simulink model "Hunter_gazebo_call"  (R2023a)
settings: Solver=ode3  StartTime=0.0  StopTime=inf  FixedStep=0.05  RelTol=1e-3  EnableMultiTasking=on
InitFcn:
  | rosshutdown
  | rosinit("http://localhost:11311")
model workspace (MAT data in the model file):
  SL_ROS_VariableLengthArrays_MaxSizes.CommonInfo.ArrayTruncateAction = 'EmitWarning'
  SL_ROS_VariableLengthArrays_MaxSizes.MsgTypeMap = containers.Map
  SL_ROS_VariableLengthArrays_MaxSizes.MsgTypeMap.serialization.keys = {'cob_object_detection_msgs/Detection', 'cob_object_detection_msgs/DetectionArray', 'gazebo_msgs/ModelStates', 'sensor_msgs/PointCloud2'}
  SL_ROS_VariableLengthArrays_MaxSizes.MsgTypeMap.serialization.values{1}(1).PropertyName = 'Detector'
  SL_ROS_VariableLengthArrays_MaxSizes.MsgTypeMap.serialization.values{1}(1).DataType = 'uint8'
  SL_ROS_VariableLengthArrays_MaxSizes.MsgTypeMap.serialization.values{1}(1).MaxLength = 128
  SL_ROS_VariableLengthArrays_MaxSizes.MsgTypeMap.serialization.values{1}(2).PropertyName = 'Label'
  SL_ROS_VariableLengthArrays_MaxSizes.MsgTypeMap.serialization.values{1}(2).DataType = 'uint8'
  SL_ROS_VariableLengthArrays_MaxSizes.MsgTypeMap.serialization.values{1}(2).MaxLength = 128
  SL_ROS_VariableLengthArrays_MaxSizes.MsgTypeMap.serialization.values{2}.PropertyName = 'Detections'
  SL_ROS_VariableLengthArrays_MaxSizes.MsgTypeMap.serialization.values{2}.DataType = 'cob_object_detection_msgs/Detection'
  SL_ROS_VariableLengthArrays_MaxSizes.MsgTypeMap.serialization.values{2}.MaxLength = 100
  SL_ROS_VariableLengthArrays_MaxSizes.MsgTypeMap.serialization.values{3}(1).PropertyName = 'Name'
  SL_ROS_VariableLengthArrays_MaxSizes.MsgTypeMap.serialization.values{3}(1).DataType = 'std_msgs/String'
  SL_ROS_VariableLengthArrays_MaxSizes.MsgTypeMap.serialization.values{3}(1).MaxLength = 266
  SL_ROS_VariableLengthArrays_MaxSizes.MsgTypeMap.serialization.values{3}(2).PropertyName = 'Pose'
  SL_ROS_VariableLengthArrays_MaxSizes.MsgTypeMap.serialization.values{3}(2).DataType = 'geometry_msgs/Pose'
  SL_ROS_VariableLengthArrays_MaxSizes.MsgTypeMap.serialization.values{3}(2).MaxLength = 350
  SL_ROS_VariableLengthArrays_MaxSizes.MsgTypeMap.serialization.values{3}(3).PropertyName = 'Twist'
  SL_ROS_VariableLengthArrays_MaxSizes.MsgTypeMap.serialization.values{3}(3).DataType = 'geometry_msgs/Twist'
  SL_ROS_VariableLengthArrays_MaxSizes.MsgTypeMap.serialization.values{3}(3).MaxLength = 350
  SL_ROS_VariableLengthArrays_MaxSizes.MsgTypeMap.serialization.values{4}(1).PropertyName = 'Data'
  SL_ROS_VariableLengthArrays_MaxSizes.MsgTypeMap.serialization.values{4}(1).DataType = 'uint8'
  SL_ROS_VariableLengthArrays_MaxSizes.MsgTypeMap.serialization.values{4}(1).MaxLength = 1050000
  SL_ROS_VariableLengthArrays_MaxSizes.MsgTypeMap.serialization.values{4}(2).PropertyName = 'Fields'
  SL_ROS_VariableLengthArrays_MaxSizes.MsgTypeMap.serialization.values{4}(2).DataType = 'sensor_msgs/PointField'
  SL_ROS_VariableLengthArrays_MaxSizes.MsgTypeMap.serialization.values{4}(2).MaxLength = 1000
  SL_ROS_VariableLengthArrays_MaxSizes.MsgTypeMap.serialization.uniformity = 0
  SL_ROS_VariableLengthArrays_MaxSizes.MsgTypeMap.serialization.keyType = 'char'
  SL_ROS_VariableLengthArrays_MaxSizes.MsgTypeMap.serialization.valueType = 'any'
values from neighbouring files (symbols this model uses):
  roi = [0, 7, -7, 7, -1, 2]    [TrackExample_sim.m]
undefined symbols (not defined in the file or in its folder): Angular, L, Ld, Linear
libraries: robotlib x20, slpidlib x4, robotalgslib x3, slctrlblks x2, mobileRoboticsLib x2, robotcorelib x2, simulink_extras x2
(part 1 of 2)
settings Model: Creator=aiv_  LastModifiedBy=aiv
settings SolverCC: AutoInsertRateTranBlk=on
settings DataIOCC: SaveFormat=Array  ReturnWorkspaceOutputs=off
settings OptimizationCC: EnhancedBackFolding=on  PassReuseOutputArgsAs=Individual arguments  StateBitsets=on  DataBitsets=on  ZeroExternalMemoryAtStartup=off  ZeroInternalMemoryAtStartup=off  NoFixptDivByZeroProtection=on  LifeSpan=1  MaxStackSize=64  OptimizeBlockOrder=speed  DifferentSizesBufferReuse=on  EfficientTunableParamExpr=on
settings DebuggingCC: ParameterTunabilityLossMsg=error
settings HardwareCC: ProdBitPerPointer=32  ProdBitPerSizeT=32  ProdBitPerPtrDiffT=32  ProdLargestAtomicFloat=None  ProdWordSize=32  ProdHWDeviceType=Custom Processor->Custom Processor
settings ModelReferenceCC: PropagateSignalLabelsOutOfModel=off
settings SFSimCC: SimTargetLang=C++
settings RTWCC: Description=Embedded Coder  SystemTargetFile=ert.tlc  HardwareBoard=Robot Operating System (ROS)  TLCOptions=-p0 -aRateBasedStepFcn=0  TemplateMakefile=ert_default_tmf  GenerateReport=on  RTWVerbose=off  Toolchain=Catkin  IncludeHyperlinkInReport=on  LaunchReport=on  TargetLang=C++
settings CodeAppCC: ForceParamTrailComments=on  IgnoreCustomStorageClasses=off  OperatorAnnotations=on  SimulinkDataObjDesc=on  SFDataObjDesc=on  CustomSymbolStrGlobalVar=rt$N$M  CustomSymbolStrType=$N$M  CustomSymbolStrFcn=$N$M$F  CustomSymbolStrMacro=$N$M  InsertBlockDesc=on
settings ERTTargetCC: CodeReplacementLibrary=GNU C99 extensions  SuppressErrorStatus=on  CodeInterfacePackaging=C++ class  SupportVariableSizeSignals=on  RootIOFormat=Structure reference  ERTCustomFileTemplate=example_file_process.tlc

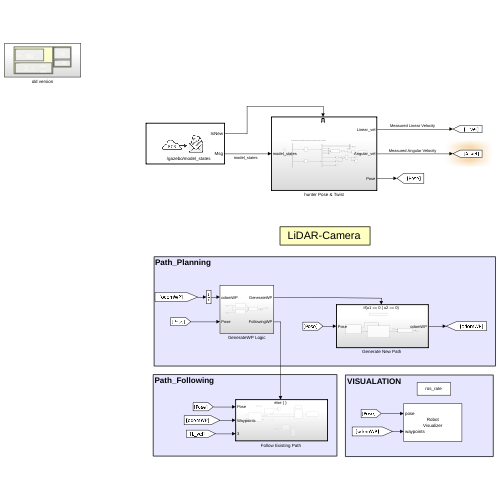
[thumbnail: Simulink's stored preview of the top-level diagram]
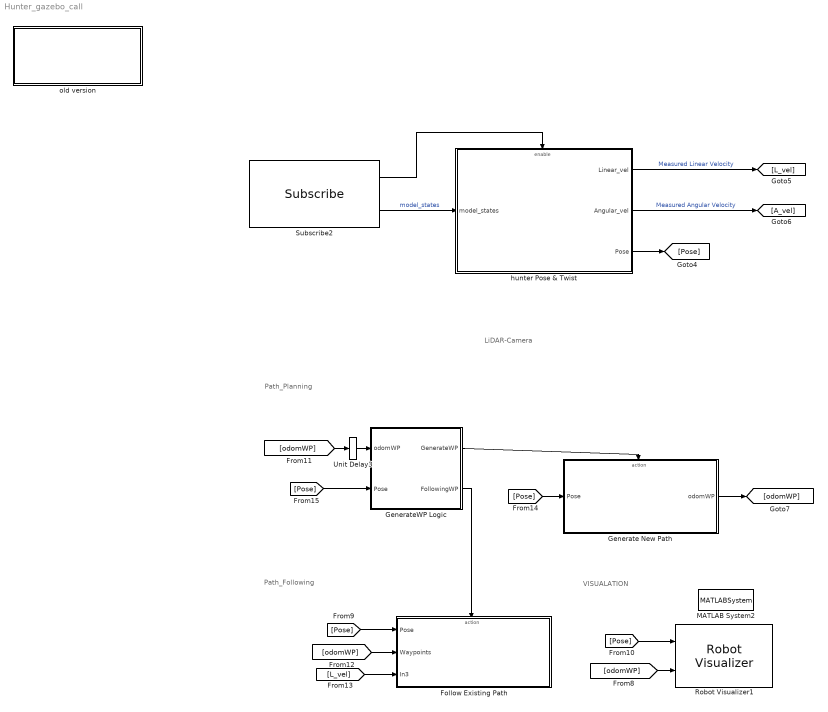
== system Hunter_gazebo_call ==
  note: LiDAR-Camera
  note: VISUALATION
  note: Path_Planning
  note: Path_Following
  "Follow Existing Path " : Subsystem  TreatAsAtomicUnit=on
  "Generate New Path " : Subsystem  TreatAsAtomicUnit=on
  GenerateWP Logic : Subsystem
  MATLAB System2 : MATLABSystem  System=ros_rate  RATE=[20]  SimulateUsing=Code generation
      mask Type: ros_rate
      mask Display: disp('ros_rate');
  Robot Visualizer1 : mobileRoboticsLib/Environments/Robot Visualizer  robotRadius=0  showTrajectory=on  hasWaypoints=on  hasLidar=off  sensorOffset=[ 0, 0 ]  scanAngles=[ -pi/4, 0, pi/4 ]  hasObjDetector=off  objDetectorOffset=[ 0, 0 ]  objDetectorAngle=0  objDetectorFOV=pi/4  objDetectorMaxRange=5  objectColors=[ 1, 0, 0; 0, 1, 0; 0, 0, 1 ]  objectMarkers=s
  Subscribe2 : robotlib/Subscribe  topicSource=Select from ROS network  topic=/gazebo/model_states  messageType=gazebo_msgs/ModelStates  SampleTime=-1  legacyBusStruct=off  messageQueueLength=1
  Unit Delay3 : UnitDelay  SampleTime=-1  HasFrameUpgradeWarning=on
  hunter Pose & Twist : Subsystem
  old version : Subsystem
  wires:
  hunter Pose & Twist/3(Pose) -> [Pose]
  Subscribe2/1 -> hunter Pose & Twist/Enable
  hunter Pose & Twist/2(Angular_vel) -> [A_vel]  "Measured Angular Velocity"
  Subscribe2/2 -> hunter Pose & Twist/1(model_states)  "model_states"
  hunter Pose & Twist/1(Linear_vel) -> [L_vel]  "Measured Linear Velocity"
  [odomWP] -> Robot Visualizer1/2
  [Pose] -> "Follow Existing Path "/1(Pose)
  "Generate New Path "/1(odomWP) -> [odomWP]
  [odomWP] -> "Follow Existing Path "/2(Waypoints)
  [Pose] -> GenerateWP Logic/2(Pose)
  [odomWP] -> Unit Delay3/1
  [Pose] -> "Generate New Path "/1(Pose)
  GenerateWP Logic/2(FollowingWP) -> "Follow Existing Path "/Action
  [Pose] -> Robot Visualizer1/1
  GenerateWP Logic/1(GenerateWP) -> "Generate New Path "/Action
  Unit Delay3/1 -> GenerateWP Logic/1(odomWP)
  [L_vel] -> "Follow Existing Path "/3(In3)

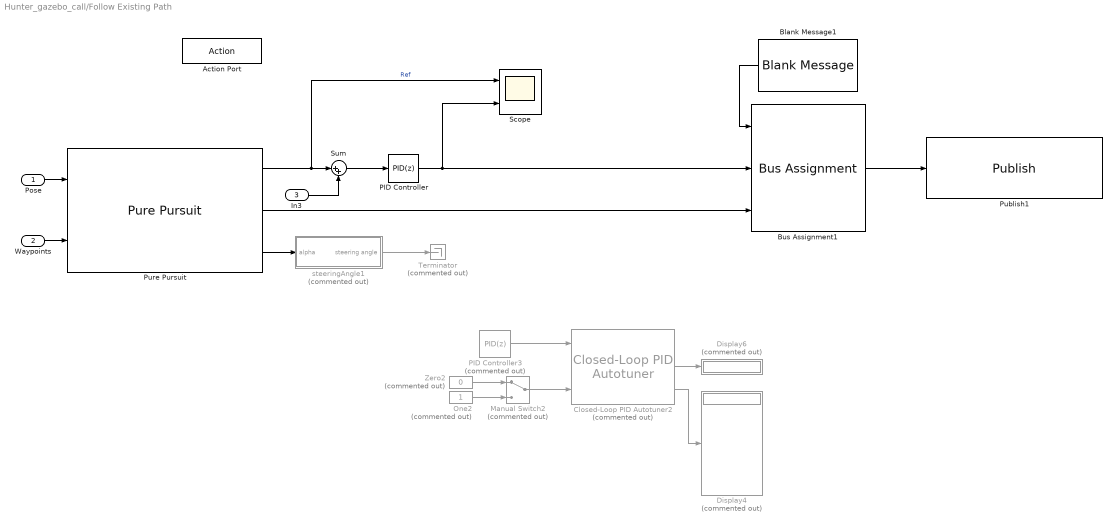
== system Hunter_gazebo_call/Follow Existing Path  ==
  Pose : Inport
  Waypoints : Inport  Port=2
  In3 : Inport  Port=3
  Action Port : ActionPort  ActionPortLabel=else
  Blank Message1 : robotlib/Blank Message  messageClass=Message  entityType=geometry_msgs/Twist  messageType=geometry_msgs/Twist  SampleTime=inf  legacyBusStruct=off
  Bus Assignment1 : BusAssignment  AssignedSignals=Linear.X,Angular.Z
  Closed-Loop PID Autotuner2 : slctrlblks/Closed-Loop PID Autotuner  Commented=on  PIDType=PID  PIDForm=Parallel  TimeDomain=discrete-time  DiscreteTs=0.05  TuningTs=0.2  UseTuningTs=off  IntegratorFormula=Forward Euler  FilterFormula=Forward Euler  ContinuousTs=0.02  Bandwidth=1  UseExternalWC=off  TargetPM=60  UseExternalPM=off  UseExternalAchievedPM=off  ExperimentMode=Superposition  PlantType=Stable  PlantSign=Positive  AmpSine=0.01  UseExternalAmpSine=off  UseExternalFRD=off  UseExternalU0=off  UseCompanion=off  NotDeployTuningModule=off  UsePLCCoder=off  OutputMode=control action + perturbation  BlockDataType=double  UseConnectedPID=on  blockpath=[]  tunedP=0  tunedI=0  tunedD=0  tunedN=100  tunedPM=0  EstimationWindowSize=3  UseExternalTuningParams=off  SingleMultiRateVariant=SingleSamplingRate  NumEstimationPeriods=4  NumSettlingPeriods=2  ExperimentModeVariant=VariantSuperimposed  OutputChoice=VariantCandD
  Display4 : Display  Commented=on
  Display6 : Display  Commented=on
  Manual Switch2 : ManualSwitch  Commented=on
  One2 : Constant  Commented=on  OutDataTypeStr=Inherit: Inherit via back propagation
  PID Controller : slpidlib/PID Controller  Controller=PID  Form=Parallel  TimeDomain=Discrete-time  UseExternalTs=off  SampleTime=-1  IntegratorMethod=Forward Euler  FilterMethod=Forward Euler  ControllerParametersSource=internal  P=0.3475  I=0.1757  UseKiTs=off  D=0  N=100  UseFilter=on  TunerSelectOption=Transfer Function Based (PID Tuner App)  InitialConditionSource=internal  InitialConditionForIntegrator=0  InitialConditionForFilter=0  DifferentiatorICPrevScaledInput=0  ExternalReset=none  TrackingMode=off  Kt=1  LimitOutput=off  SatLimitsSource=internal  UpperSaturationLimit=inf  LowerSaturationLimit=-inf  LinearizeAsGain=on  AntiWindupMode=none  Kb=1  LimitIntegrator=off  UpperIntegratorSaturationLimit=inf  LowerIntegratorSaturationLimit=-inf  POutMin=[]  POutMax=[]  IOutMin=[]  IOutMax=[]  DOutMin=[]  DOutMax=[]  NOutMin=[]  NOutMax=[]  SumOutMin=[]  SumOutMax=[]  SaturationOutMin=[]  SaturationOutMax=[]  PParamMin=[]  PParamMax=[]  IParamMin=[]  IParamMax=[]  DParamMin=[]  DParamMax=[]  NParamMin=[]  NParamMax=[]  KbParamMin=[]  KbParamMax=[]  KtParamMin=[]  KtParamMax=[]  KbOutMin=[]  KbOutMax=[]  KtOutMin=[]  KtOutMax=[]  IntegratorOutMin=[]  IntegratorOutMax=[]  FilterOutMin=[]  FilterOutMax=[]  SumI1OutMin=[]  SumI1OutMax=[]  SumI2OutMin=[]  SumI2OutMax=[]  SumI3OutMin=[]  SumI3OutMax=[]  SumI4OutMin=[]  SumI4OutMax=[]  SumDOutMin=[]  SumDOutMax=[]  DifferentiatorOutMin=[]  DifferentiatorOutMax=[]  FilterDiffOutCoefMin=[]  FilterDiffOutCoefMax=[]  ReciprocalOutMin=[]  ReciprocalOutMax=[]  SumDenOutMin=[]  SumDenOutMax=[]  SumNumOutMin=[]  SumNumOutMax=[]  DivideOutMin=[]  DivideOutMax=[]  UdiffTsProdOutMin=[]  UdiffTsProdOutMax=[]  NTsProdOutMin=[]  NTsProdOutMax=[]  UintegralTsProdOutMin=[]  UintegralTsProdOutMax=[]  UngainTsProdOutMin=[]  UngainTsProdOutMax=[]  ClampingZeroOutDataTypeStr=Inherit: Inherit via back propagation  ClampingZeroOutMin=[]  ClampingZeroOutMax=[]  FilterDenConstantOutDataTypeStr=Inherit: Inherit via back propagation  FilterDenConstantOutMin=[]  FilterDenConstantOutMax=[]  PCopyOutDataTypeStr=Inherit: Inherit via back propagation  PCopyOutMin=[]  PCopyOutMax=[]  NCopyOutDataTypeStr=Inherit: Inherit via back propagation  NCopyOutMin=[]  NCopyOutMax=[]  IntegratorContinuousStateAttributes=''  IntegratorStateMustResolveToSignalObject=off  IntegratorRTWStateStorageClass=Auto  FilterContinuousStateAttributes=''  FilterStateMustResolveToSignalObject=off  FilterRTWStateStorageClass=Auto  ParallelPVariant=InternalParameters  IdealPVariant=Disabled  IVariant=InternalParameters  DVariant=InternalParameters  IntegratorVariant=Discrete  SatVariant=Disabled  AWVariant=Passthrough  PCopyVariant=Disabled  TRVariant=Disabled  FdbkBlocksVariant=Forward  IdealPFdbkVariant=Disabled  SatFdbkVariant=Disabled  DerivativeFilterVariant=ForwardEulerFilter  NVariant=InternalParameters  NCopyVariant=Disabled  FilterICVariant=InternalICsFilter  IntegratorICVariant=InternalICs  ExternalResetVariant=Disabled  TRSumVariant=Passthrough  SumFdbkVariant=Disabled  SumVariant=Sum_PID  TsampFilterVariant=InternalTs  TsampNgainVariant=Passthrough  TsampIntegralVariant=Disabled_SignalSpec  ExternalSaturationOutDataTypeStr=Inherit: Same as second input
  PID Controller3 : slpidlib/PID Controller  Commented=on  Controller=PID  Form=Parallel  TimeDomain=Discrete-time  UseExternalTs=off  SampleTime=-1  IntegratorMethod=Forward Euler  FilterMethod=Forward Euler  ControllerParametersSource=internal  P=1  I=1  UseKiTs=off  D=0  N=100  UseFilter=on  TunerSelectOption=Transfer Function Based (PID Tuner App)  InitialConditionSource=internal  InitialConditionForIntegrator=0  InitialConditionForFilter=0  DifferentiatorICPrevScaledInput=0  ExternalReset=none  TrackingMode=off  Kt=1  LimitOutput=off  SatLimitsSource=internal  UpperSaturationLimit=inf  LowerSaturationLimit=-inf  LinearizeAsGain=on  AntiWindupMode=none  Kb=1  LimitIntegrator=off  UpperIntegratorSaturationLimit=inf  LowerIntegratorSaturationLimit=-inf  POutMin=[]  POutMax=[]  IOutMin=[]  IOutMax=[]  DOutMin=[]  DOutMax=[]  NOutMin=[]  NOutMax=[]  SumOutMin=[]  SumOutMax=[]  SaturationOutMin=[]  SaturationOutMax=[]  PParamMin=[]  PParamMax=[]  IParamMin=[]  IParamMax=[]  DParamMin=[]  DParamMax=[]  NParamMin=[]  NParamMax=[]  KbParamMin=[]  KbParamMax=[]  KtParamMin=[]  KtParamMax=[]  KbOutMin=[]  KbOutMax=[]  KtOutMin=[]  KtOutMax=[]  IntegratorOutMin=[]  IntegratorOutMax=[]  FilterOutMin=[]  FilterOutMax=[]  SumI1OutMin=[]  SumI1OutMax=[]  SumI2OutMin=[]  SumI2OutMax=[]  SumI3OutMin=[]  SumI3OutMax=[]  SumI4OutMin=[]  SumI4OutMax=[]  SumDOutMin=[]  SumDOutMax=[]  DifferentiatorOutMin=[]  DifferentiatorOutMax=[]  FilterDiffOutCoefMin=[]  FilterDiffOutCoefMax=[]  ReciprocalOutMin=[]  ReciprocalOutMax=[]  SumDenOutMin=[]  SumDenOutMax=[]  SumNumOutMin=[]  SumNumOutMax=[]  DivideOutMin=[]  DivideOutMax=[]  UdiffTsProdOutMin=[]  UdiffTsProdOutMax=[]  NTsProdOutMin=[]  NTsProdOutMax=[]  UintegralTsProdOutMin=[]  UintegralTsProdOutMax=[]  UngainTsProdOutMin=[]  UngainTsProdOutMax=[]  ClampingZeroOutDataTypeStr=Inherit: Inherit via back propagation  ClampingZeroOutMin=[]  ClampingZeroOutMax=[]  FilterDenConstantOutDataTypeStr=Inherit: Inherit via back propagation  FilterDenConstantOutMin=[]  FilterDenConstantOutMax=[]  PCopyOutDataTypeStr=Inherit: Inherit via back propagation  PCopyOutMin=[]  PCopyOutMax=[]  NCopyOutDataTypeStr=Inherit: Inherit via back propagation  NCopyOutMin=[]  NCopyOutMax=[]  IntegratorContinuousStateAttributes=''  IntegratorStateMustResolveToSignalObject=off  IntegratorRTWStateStorageClass=Auto  FilterContinuousStateAttributes=''  FilterStateMustResolveToSignalObject=off  FilterRTWStateStorageClass=Auto  ParallelPVariant=InternalParameters  IdealPVariant=Disabled  IVariant=InternalParameters  DVariant=InternalParameters  IntegratorVariant=Discrete  SatVariant=Disabled  AWVariant=Passthrough  PCopyVariant=Disabled  TRVariant=Disabled  FdbkBlocksVariant=Forward  IdealPFdbkVariant=Disabled  SatFdbkVariant=Disabled  DerivativeFilterVariant=ForwardEulerFilter  NVariant=InternalParameters  NCopyVariant=Disabled  FilterICVariant=InternalICsFilter  IntegratorICVariant=InternalICs  ExternalResetVariant=Disabled  TRSumVariant=Passthrough  SumFdbkVariant=Disabled  SumVariant=Sum_PID  TsampFilterVariant=InternalTs  TsampNgainVariant=Passthrough  TsampIntegralVariant=Disabled_SignalSpec  ExternalSaturationOutDataTypeStr=Inherit: Same as second input
  Publish1 : robotlib/Publish  topicSource=Select from ROS network  topic=/ackermann_steering_controller/cmd_vel  messageType=geometry_msgs/Twist  legacyBusStruct=off  messageQueueLength=1
  Pure Pursuit : robotalgslib/Pure Pursuit  DesiredLinearVelocity=1.5  MaxAngularVelocity=2  LookaheadDistance=1.3  TargetDirPort=on  SimulateUsing=Code generation
      settings: LibrarySourceBlock=navlib/Control Algorithms/Pure Pursuit
  Scope : Scope  NumInputPorts=2
  Sum : Sum  Inputs=|++
  Terminator : Terminator  Commented=on
  Zero2 : Constant  Commented=on  Value=0  OutDataTypeStr=Inherit: Inherit via back propagation
  steeringAngle1 : Subsystem  Commented=on
  wires:
  Pose/1 -> Pure Pursuit/1
  Waypoints/1 -> Pure Pursuit/2
  Bus Assignment1/1 -> Publish1/1
  Blank Message1/1 -> Bus Assignment1/1
  Pure Pursuit/3 -> steeringAngle1/1(alpha)
  Pure Pursuit/2 -> Bus Assignment1/3
  PID Controller/1 -> Scope/2, Bus Assignment1/2
  Sum/1 -> PID Controller/1
  Pure Pursuit/1 -> Scope/1, Sum/1  "Ref"
  In3/1 -> Sum/2
  PID Controller3/1 -> Closed-Loop PID Autotuner2/1
  Manual Switch2/1 -> Closed-Loop PID Autotuner2/3
  Closed-Loop PID Autotuner2/3 -> Display4/1
  Zero2/1 -> Manual Switch2/1
  Closed-Loop PID Autotuner2/2 -> Display6/1
  One2/1 -> Manual Switch2/2
  steeringAngle1/1(steering angle) -> Terminator/1

== system Hunter_gazebo_call/Generate New Path  ==
  Pose : Inport
  Action Port : ActionPort  PropagateVarSize=During execution  ActionPortLabel=if(u1 == 0 | u2 == 0)
  Generate New Waypoint : Subsystem
  Subscribe : robotlib/Subscribe  topicSource=Select from ROS network  topic=/lidar  messageType=sensor_msgs/PointCloud2  SampleTime=-1  legacyBusStruct=off  messageQueueLength=1
  generate_odomWaypoints : MATLAB Function  TreatAsAtomicUnit=on
  odomWP : Outport
  wires:
  Subscribe/2 -> Generate New Waypoint/1(rawData)
  generate_odomWaypoints/1(odomWaypoints) -> odomWP/1
  Subscribe/1 -> Generate New Waypoint/Enable
  Pose/1 -> generate_odomWaypoints/1(pose)
  Generate New Waypoint/1(waypoints) -> generate_odomWaypoints/2(waypoints)

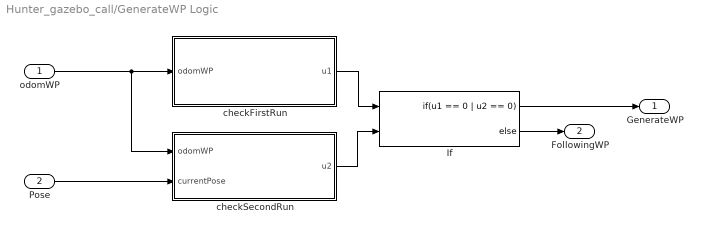
== system Hunter_gazebo_call/GenerateWP Logic ==
  odomWP : Inport
  Pose : Inport  Port=2
  If : If  NumInputs=2  IfExpression=u1 == 0 | u2 == 0
  checkFirstRun : MATLAB Function  TreatAsAtomicUnit=on
  checkSecondRun : MATLAB Function  TreatAsAtomicUnit=on
  GenerateWP : Outport
  FollowingWP : Outport  Port=2
  wires:
  checkSecondRun/1(u2) -> If/2
  odomWP/1 -> checkSecondRun/1(odomWP), checkFirstRun/1(odomWP)
  If/2 -> FollowingWP/1
  checkFirstRun/1(u1) -> If/1
  Pose/1 -> checkSecondRun/2(currentPose)
  If/1 -> GenerateWP/1

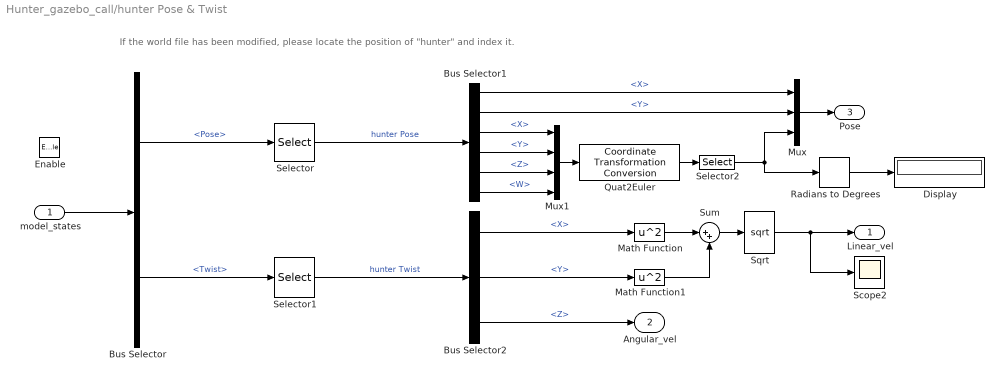
== system Hunter_gazebo_call/hunter Pose & Twist ==
  note: If the world file has been modified, please locate the position of "hunter" and index it.
  model_states : Inport
  Enable : EnablePort  StatesWhenEnabling=reset
  Bus Selector : BusSelector  OutputSignals=Pose,Twist
  Bus Selector1 : BusSelector  OutputSignals=Position.X,Position.Y,Orientation.X,Orientation.Y,Orientation.Z,Orientation.W
  Bus Selector2 : BusSelector  OutputSignals=Linear.X,Linear.Y,Angular.Z
  Display : Display
  Math Function : Math  Operator=square
  Math Function1 : Math  Operator=square
  Mux : Mux  Inputs=3
  Mux1 : Mux
  Quat2Euler : robotcorelib/Coordinate Transformation Conversion  InputRepresentation=Quaternion  InputEulerSequence=ZYX  ShowTrVecInputPort=on  OutputRepresentation=Euler Angles  OutputEulerSequence=ZYX  ShowTrVecOutputPort=on  SimulateUsing=Interpreted execution
  Radians to Degrees : simulink_extras/Transformations/Radians to Degrees
  Scope2 : Scope
  Selector : Selector  InputPortWidth=350  IndexOptions=Index vector (dialog)  Indices=[137]  OutputSizes=1
  Selector1 : Selector  InputPortWidth=350  IndexOptions=Index vector (dialog)  Indices=[137]  OutputSizes=1
  Selector2 : Selector  InputPortWidth=3  IndexOptions=Index vector (dialog)  Indices=3  OutputSizes=1
  Sqrt : Sqrt
  Sum : Sum  Inputs=|++
  Linear_vel : Outport
  Angular_vel : Outport  Port=2
  Pose : Outport  Port=3
  wires:
  model_states/1 -> Bus Selector/1
  Bus Selector1/5 -> Mux1/3  "<Z>"
  Bus Selector1/3 -> Mux1/1  "<X>"
  Selector/1 -> Bus Selector1/1  "hunter Pose"
  Bus Selector1/6 -> Mux1/4  "<W>"
  Bus Selector2/1 -> Math Function/1  "<X>"
  Bus Selector1/4 -> Mux1/2  "<Y>"
  Selector1/1 -> Bus Selector2/1  "hunter Twist"
  Bus Selector1/1 -> Mux/1  "<X>"
  Bus Selector1/2 -> Mux/2  "<Y>"
  Bus Selector/1 -> Selector/1  "<Pose>"
  Bus Selector/2 -> Selector1/1  "<Twist>"
  Selector2/1 -> Mux/3, Radians to Degrees/1
  Sum/1 -> Sqrt/1
  Bus Selector2/2 -> Math Function1/1  "<Y>"
  Math Function/1 -> Sum/1
  Math Function1/1 -> Sum/2
  Sqrt/1 -> Linear_vel/1, Scope2/1
  Bus Selector2/3 -> Angular_vel/1  "<Z>"
  Mux/1 -> Pose/1
  Mux1/1 -> Quat2Euler/1
  Quat2Euler/1 -> Selector2/1
  Radians to Degrees/1 -> Display/1

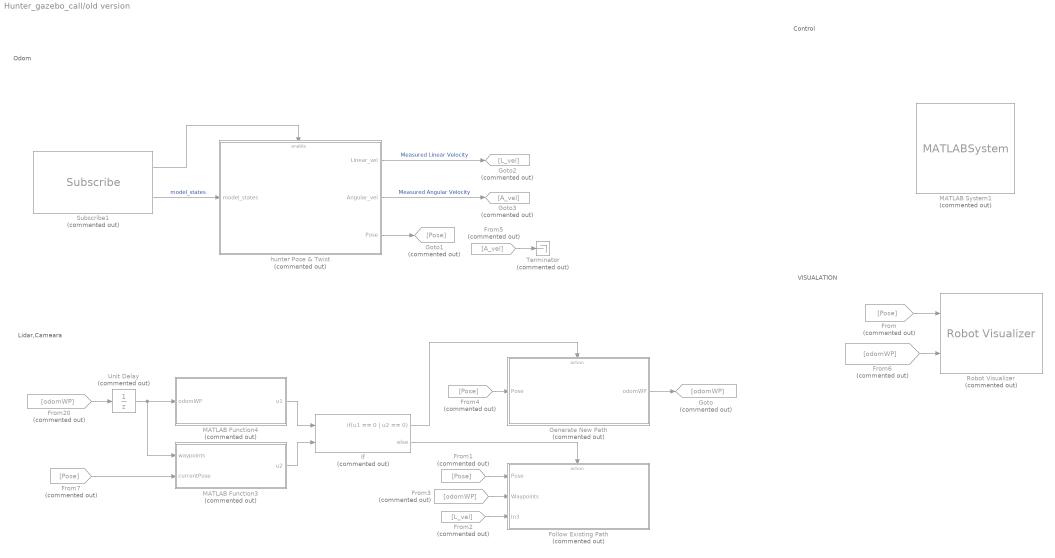
== system Hunter_gazebo_call/old version ==
  note: VISUALATION
  note: Odom
  note: Control
  note: Lidar,Cameara
  "Follow Existing Path " : Subsystem  Commented=on  TreatAsAtomicUnit=on
  From{,1,4,7} (4 alike) : From  Commented=on  GotoTag=Pose
  From2 : From  Commented=on  GotoTag=L_vel
  From20 : From  Commented=on  GotoTag=odomWP
  From3 : From  Commented=on  GotoTag=odomWP
  From5 : From  Commented=on  GotoTag=A_vel
  From6 : From  Commented=on  GotoTag=odomWP
  "Generate New Path " : Subsystem  Commented=on  TreatAsAtomicUnit=on
  Goto : Goto  Commented=on  GotoTag=odomWP
  Goto1 : Goto  Commented=on  GotoTag=Pose
  Goto2 : Goto  Commented=on  GotoTag=L_vel
  Goto3 : Goto  Commented=on  GotoTag=A_vel
  If : If  Commented=on  NumInputs=2  IfExpression=u1 == 0 | u2 == 0
  MATLAB Function3 : MATLAB Function  Commented=on  TreatAsAtomicUnit=on
  MATLAB Function4 : MATLAB Function  Commented=on  TreatAsAtomicUnit=on
  MATLAB System1 : MATLABSystem  Commented=on  System=ros_rate  RATE=[20]  SimulateUsing=Code generation
      mask Type: ros_rate
      mask Display: disp('ros_rate');
  Robot Visualizer : mobileRoboticsLib/Environments/Robot Visualizer  Commented=on  robotRadius=0  showTrajectory=on  hasWaypoints=on  hasLidar=off  sensorOffset=[ 0, 0 ]  scanAngles=[ -pi/4, 0, pi/4 ]  hasObjDetector=off  objDetectorOffset=[ 0, 0 ]  objDetectorAngle=0  objDetectorFOV=pi/4  objDetectorMaxRange=5  objectColors=[ 1, 0, 0; 0, 1, 0; 0, 0, 1 ]  objectMarkers=s
  Subscribe1 : robotlib/Subscribe  Commented=on  topicSource=Select from ROS network  topic=/gazebo/model_states  messageType=gazebo_msgs/ModelStates  SampleTime=-1  legacyBusStruct=off  messageQueueLength=1
  Terminator : Terminator  Commented=on
  Unit Delay : UnitDelay  Commented=on  SampleTime=-1  HasFrameUpgradeWarning=on
  hunter Pose & Twist : Subsystem  Commented=on
  wires:
  MATLAB Function4/1(u1) -> If/1
  From1/1 -> "Follow Existing Path "/1(Pose)
  If/2 -> "Follow Existing Path "/Action
  From20/1 -> Unit Delay/1
  From/1 -> Robot Visualizer/1
  hunter Pose & Twist/2(Angular_vel) -> Goto3/1  "Measured Angular Velocity"
  hunter Pose & Twist/3(Pose) -> Goto1/1
  Subscribe1/2 -> hunter Pose & Twist/1(model_states)  "model_states"
  From2/1 -> "Follow Existing Path "/3(In3)
  From3/1 -> "Follow Existing Path "/2(Waypoints)
  MATLAB Function3/1(u2) -> If/2
  If/1 -> "Generate New Path "/Action
  Subscribe1/1 -> hunter Pose & Twist/Enable
  "Generate New Path "/1(odomWP) -> Goto/1
  From6/1 -> Robot Visualizer/2
  From7/1 -> MATLAB Function3/2(currentPose)
  Unit Delay/1 -> MATLAB Function3/1(waypoints), MATLAB Function4/1(odomWP)
  From5/1 -> Terminator/1
  From4/1 -> "Generate New Path "/1(Pose)
  hunter Pose & Twist/1(Linear_vel) -> Goto2/1  "Measured Linear Velocity"

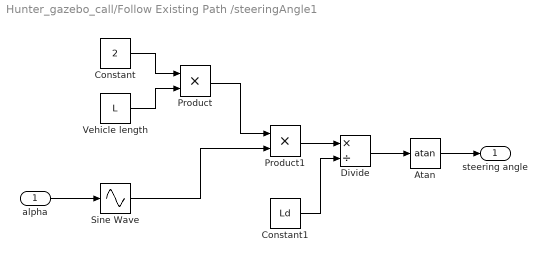
== system Hunter_gazebo_call/Follow Existing Path /steeringAngle1 ==
  alpha : Inport
  Atan : Trigonometry  Operator=atan
  Constant : Constant  Value=2
  Constant1 : Constant  Value=Ld
  Divide : Product  Inputs=*/
  Product : Product
  Product1 : Product
  Sine Wave : Sin  TimeSource=Use external signal  SampleTime=0
  Vehicle length : Constant  Value=L
  steering angle : Outport
  wires:
  Constant/1 -> Product/1
  Vehicle length/1 -> Product/2
  alpha/1 -> Sine Wave/1
  Product/1 -> Product1/1
  Sine Wave/1 -> Product1/2
  Product1/1 -> Divide/1
  Constant1/1 -> Divide/2
  Divide/1 -> Atan/1
  Atan/1 -> steering angle/1

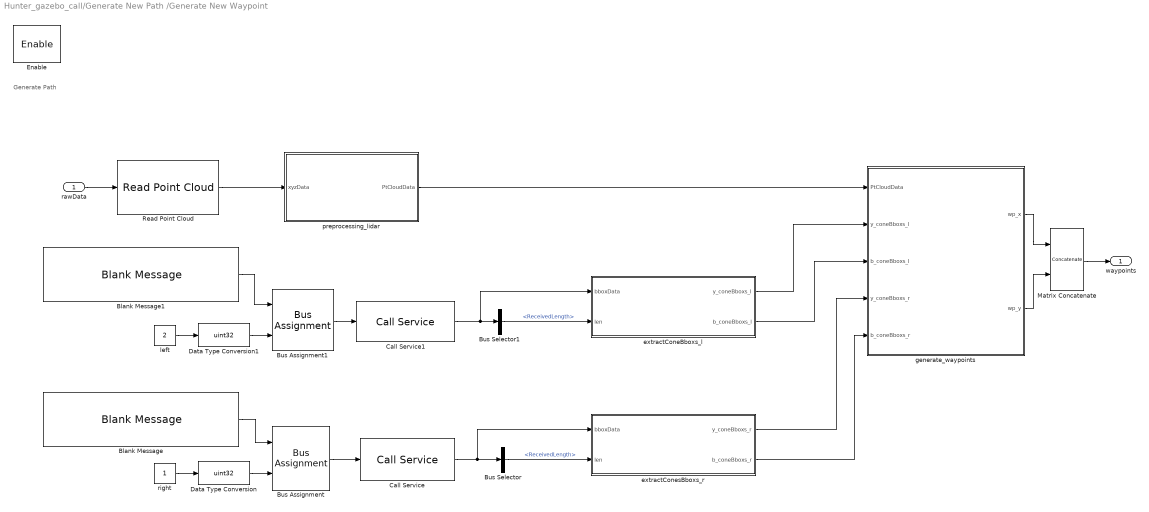
== system Hunter_gazebo_call/Generate New Path /Generate New Waypoint ==
  note: Generate Path
  rawData : Inport
  Enable : EnablePort  PropagateVarSize=During execution
  Blank Message : robotlib/Blank Message  messageClass=Service Request  entityType=cob_object_detection_msgs/DetectObjects  messageType=cob_object_detection_msgs/DetectObjectsRequest  SampleTime=inf  legacyBusStruct=off
  Blank Message1 : robotlib/Blank Message  messageClass=Service Request  entityType=cob_object_detection_msgs/DetectObjects  messageType=cob_object_detection_msgs/DetectObjectsRequest  SampleTime=inf  legacyBusStruct=off
  Bus Assignment : BusAssignment  AssignedSignals=Roi.Height
  Bus Assignment1 : BusAssignment  AssignedSignals=Roi.Height
  Bus Selector : BusSelector  OutputSignals=ObjectList.Detections_SL_Info.ReceivedLength
  Bus Selector1 : BusSelector  OutputSignals=ObjectList.Detections_SL_Info.ReceivedLength
  Call Service : robotlib/Call Service  topicSource=Specify your own  service=/Activate_yolo  serviceType=cob_object_detection_msgs/DetectObjects  connectionTimeout=5  keepPersistent=off  ShowErrorCodeOutput=off  legacyBusStruct=off
  Call Service1 : robotlib/Call Service  topicSource=Specify your own  service=/Activate_yolo  serviceType=cob_object_detection_msgs/DetectObjects  connectionTimeout=5  keepPersistent=off  ShowErrorCodeOutput=off  legacyBusStruct=off
  Data Type Conversion : DataTypeConversion  OutDataTypeStr=uint32  SaturateOnIntegerOverflow=off  RndMeth=Floor
  Data Type Conversion1 : DataTypeConversion  OutDataTypeStr=uint32  SaturateOnIntegerOverflow=off  RndMeth=Floor
  Matrix Concatenate : Concatenate  Mode=Multidimensional array  ConcatenateDimension=2
  Read Point Cloud : robotlib/Read Point Cloud  MaximumPointCloudSize=[1, 32768]  PreserveStructure=on  ShowRGBOutput=off  ShowIntensityOutput=off  ShowErrorCodeOutput=off  VariableSizeOutputs=off
  extractConeBboxs_l : MATLAB Function  TreatAsAtomicUnit=on
  extractConesBboxs_r : MATLAB Function  TreatAsAtomicUnit=on
  generate_waypoints : MATLAB Function  TreatAsAtomicUnit=on
  left : Constant  Value=2
  preprocessing_lidar : MATLAB Function  TreatAsAtomicUnit=on
  right : Constant
  waypoints : Outport
  wires:
  rawData/1 -> Read Point Cloud/1
  Read Point Cloud/1 -> preprocessing_lidar/1(xyzData)
  Call Service/1 -> Bus Selector/1, extractConesBboxs_r/1(bboxData)
  right/1 -> Data Type Conversion/1
  Bus Assignment1/1 -> Call Service1/1
  Data Type Conversion/1 -> Bus Assignment/2
  Blank Message1/1 -> Bus Assignment1/1
  left/1 -> Data Type Conversion1/1
  Call Service1/1 -> extractConeBboxs_l/1(bboxData), Bus Selector1/1
  Bus Selector1/1 -> extractConeBboxs_l/2(len)  "<ReceivedLength>"
  Bus Selector/1 -> extractConesBboxs_r/2(len)  "<ReceivedLength>"
  Bus Assignment/1 -> Call Service/1
  Data Type Conversion1/1 -> Bus Assignment1/2
  Blank Message/1 -> Bus Assignment/1
  extractConeBboxs_l/1(y_coneBboxs_l) -> generate_waypoints/2(y_coneBboxs_l)
  extractConeBboxs_l/2(b_coneBboxs_l) -> generate_waypoints/3(b_coneBboxs_l)
  preprocessing_lidar/1(PtCloudData) -> generate_waypoints/1(PtCloudData)
  extractConesBboxs_r/1(y_coneBboxs_r) -> generate_waypoints/4(y_coneBboxs_r)
  extractConesBboxs_r/2(b_coneBboxs_r) -> generate_waypoints/5(b_coneBboxs_r)
  generate_waypoints/1(wp_x) -> Matrix Concatenate/1
  generate_waypoints/2(wp_y) -> Matrix Concatenate/2
  Matrix Concatenate/1 -> waypoints/1

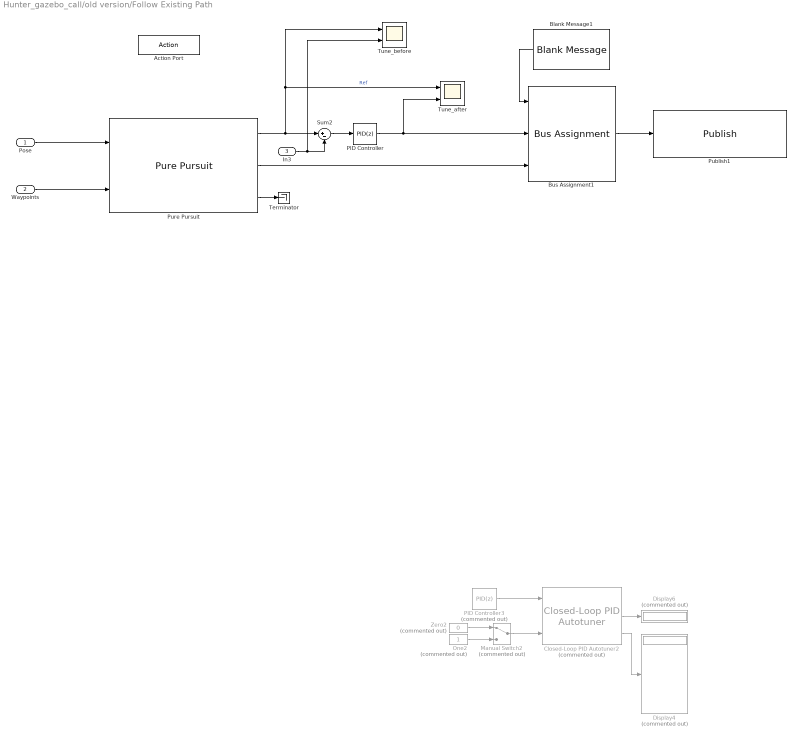
== system Hunter_gazebo_call/old version/Follow Existing Path  ==
  Pose : Inport
  Waypoints : Inport  Port=2
  In3 : Inport  Port=3
  Action Port : ActionPort  ActionPortLabel=else
  Blank Message1 : robotlib/Blank Message  messageClass=Message  entityType=geometry_msgs/Twist  messageType=geometry_msgs/Twist  SampleTime=inf  legacyBusStruct=off
  Bus Assignment1 : BusAssignment  AssignedSignals=Linear.X,Angular.Z
  Closed-Loop PID Autotuner2 : slctrlblks/Closed-Loop PID Autotuner  Commented=on  PIDType=PID  PIDForm=Parallel  TimeDomain=discrete-time  DiscreteTs=0.05  TuningTs=0.2  UseTuningTs=off  IntegratorFormula=Forward Euler  FilterFormula=Forward Euler  ContinuousTs=0.02  Bandwidth=1  UseExternalWC=off  TargetPM=60  UseExternalPM=off  UseExternalAchievedPM=off  ExperimentMode=Superposition  PlantType=Stable  PlantSign=Positive  AmpSine=0.01  UseExternalAmpSine=off  UseExternalFRD=off  UseExternalU0=off  UseCompanion=off  NotDeployTuningModule=off  UsePLCCoder=off  OutputMode=control action + perturbation  BlockDataType=double  UseConnectedPID=on  blockpath=[]  tunedP=0  tunedI=0  tunedD=0  tunedN=100  tunedPM=0  EstimationWindowSize=3  UseExternalTuningParams=off  SingleMultiRateVariant=SingleSamplingRate  NumEstimationPeriods=4  NumSettlingPeriods=2  ExperimentModeVariant=VariantSuperimposed  OutputChoice=VariantCandD
  Display4 : Display  Commented=on
  Display6 : Display  Commented=on
  Manual Switch2 : ManualSwitch  Commented=on
  One2 : Constant  Commented=on  OutDataTypeStr=Inherit: Inherit via back propagation
  PID Controller : slpidlib/PID Controller  Controller=PID  Form=Parallel  TimeDomain=Discrete-time  UseExternalTs=off  SampleTime=-1  IntegratorMethod=Forward Euler  FilterMethod=Forward Euler  ControllerParametersSource=internal  P=0.3475  I=0.1757  UseKiTs=off  D=0  N=100  UseFilter=on  TunerSelectOption=Transfer Function Based (PID Tuner App)  InitialConditionSource=internal  InitialConditionForIntegrator=0  InitialConditionForFilter=0  DifferentiatorICPrevScaledInput=0  ExternalReset=none  TrackingMode=off  Kt=1  LimitOutput=off  SatLimitsSource=internal  UpperSaturationLimit=inf  LowerSaturationLimit=-inf  LinearizeAsGain=on  AntiWindupMode=none  Kb=1  LimitIntegrator=off  UpperIntegratorSaturationLimit=inf  LowerIntegratorSaturationLimit=-inf  POutMin=[]  POutMax=[]  IOutMin=[]  IOutMax=[]  DOutMin=[]  DOutMax=[]  NOutMin=[]  NOutMax=[]  SumOutMin=[]  SumOutMax=[]  SaturationOutMin=[]  SaturationOutMax=[]  PParamMin=[]  PParamMax=[]  IParamMin=[]  IParamMax=[]  DParamMin=[]  DParamMax=[]  NParamMin=[]  NParamMax=[]  KbParamMin=[]  KbParamMax=[]  KtParamMin=[]  KtParamMax=[]  KbOutMin=[]  KbOutMax=[]  KtOutMin=[]  KtOutMax=[]  IntegratorOutMin=[]  IntegratorOutMax=[]  FilterOutMin=[]  FilterOutMax=[]  SumI1OutMin=[]  SumI1OutMax=[]  SumI2OutMin=[]  SumI2OutMax=[]  SumI3OutMin=[]  SumI3OutMax=[]  SumI4OutMin=[]  SumI4OutMax=[]  SumDOutMin=[]  SumDOutMax=[]  DifferentiatorOutMin=[]  DifferentiatorOutMax=[]  FilterDiffOutCoefMin=[]  FilterDiffOutCoefMax=[]  ReciprocalOutMin=[]  ReciprocalOutMax=[]  SumDenOutMin=[]  SumDenOutMax=[]  SumNumOutMin=[]  SumNumOutMax=[]  DivideOutMin=[]  DivideOutMax=[]  UdiffTsProdOutMin=[]  UdiffTsProdOutMax=[]  NTsProdOutMin=[]  NTsProdOutMax=[]  UintegralTsProdOutMin=[]  UintegralTsProdOutMax=[]  UngainTsProdOutMin=[]  UngainTsProdOutMax=[]  ClampingZeroOutDataTypeStr=Inherit: Inherit via back propagation  ClampingZeroOutMin=[]  ClampingZeroOutMax=[]  FilterDenConstantOutDataTypeStr=Inherit: Inherit via back propagation  FilterDenConstantOutMin=[]  FilterDenConstantOutMax=[]  PCopyOutDataTypeStr=Inherit: Inherit via back propagation  PCopyOutMin=[]  PCopyOutMax=[]  NCopyOutDataTypeStr=Inherit: Inherit via back propagation  NCopyOutMin=[]  NCopyOutMax=[]  IntegratorContinuousStateAttributes=''  IntegratorStateMustResolveToSignalObject=off  IntegratorRTWStateStorageClass=Auto  FilterContinuousStateAttributes=''  FilterStateMustResolveToSignalObject=off  FilterRTWStateStorageClass=Auto  ParallelPVariant=InternalParameters  IdealPVariant=Disabled  IVariant=InternalParameters  DVariant=InternalParameters  IntegratorVariant=Discrete  SatVariant=Disabled  AWVariant=Passthrough  PCopyVariant=Disabled  TRVariant=Disabled  FdbkBlocksVariant=Forward  IdealPFdbkVariant=Disabled  SatFdbkVariant=Disabled  DerivativeFilterVariant=ForwardEulerFilter  NVariant=InternalParameters  NCopyVariant=Disabled  FilterICVariant=InternalICsFilter  IntegratorICVariant=InternalICs  ExternalResetVariant=Disabled  TRSumVariant=Passthrough  SumFdbkVariant=Disabled  SumVariant=Sum_PID  TsampFilterVariant=InternalTs  TsampNgainVariant=Passthrough  TsampIntegralVariant=Disabled_SignalSpec  ExternalSaturationOutDataTypeStr=Inherit: Same as second input
  PID Controller3 : slpidlib/PID Controller  Commented=on  Controller=PID  Form=Parallel  TimeDomain=Discrete-time  UseExternalTs=off  SampleTime=-1  IntegratorMethod=Forward Euler  FilterMethod=Forward Euler  ControllerParametersSource=internal  P=1  I=1  UseKiTs=off  D=0  N=100  UseFilter=on  TunerSelectOption=Transfer Function Based (PID Tuner App)  InitialConditionSource=internal  InitialConditionForIntegrator=0  InitialConditionForFilter=0  DifferentiatorICPrevScaledInput=0  ExternalReset=none  TrackingMode=off  Kt=1  LimitOutput=off  SatLimitsSource=internal  UpperSaturationLimit=inf  LowerSaturationLimit=-inf  LinearizeAsGain=on  AntiWindupMode=none  Kb=1  LimitIntegrator=off  UpperIntegratorSaturationLimit=inf  LowerIntegratorSaturationLimit=-inf  POutMin=[]  POutMax=[]  IOutMin=[]  IOutMax=[]  DOutMin=[]  DOutMax=[]  NOutMin=[]  NOutMax=[]  SumOutMin=[]  SumOutMax=[]  SaturationOutMin=[]  SaturationOutMax=[]  PParamMin=[]  PParamMax=[]  IParamMin=[]  IParamMax=[]  DParamMin=[]  DParamMax=[]  NParamMin=[]  NParamMax=[]  KbParamMin=[]  KbParamMax=[]  KtParamMin=[]  KtParamMax=[]  KbOutMin=[]  KbOutMax=[]  KtOutMin=[]  KtOutMax=[]  IntegratorOutMin=[]  IntegratorOutMax=[]  FilterOutMin=[]  FilterOutMax=[]  SumI1OutMin=[]  SumI1OutMax=[]  SumI2OutMin=[]  SumI2OutMax=[]  SumI3OutMin=[]  SumI3OutMax=[]  SumI4OutMin=[]  SumI4OutMax=[]  SumDOutMin=[]  SumDOutMax=[]  DifferentiatorOutMin=[]  DifferentiatorOutMax=[]  FilterDiffOutCoefMin=[]  FilterDiffOutCoefMax=[]  ReciprocalOutMin=[]  ReciprocalOutMax=[]  SumDenOutMin=[]  SumDenOutMax=[]  SumNumOutMin=[]  SumNumOutMax=[]  DivideOutMin=[]  DivideOutMax=[]  UdiffTsProdOutMin=[]  UdiffTsProdOutMax=[]  NTsProdOutMin=[]  NTsProdOutMax=[]  UintegralTsProdOutMin=[]  UintegralTsProdOutMax=[]  UngainTsProdOutMin=[]  UngainTsProdOutMax=[]  ClampingZeroOutDataTypeStr=Inherit: Inherit via back propagation  ClampingZeroOutMin=[]  ClampingZeroOutMax=[]  FilterDenConstantOutDataTypeStr=Inherit: Inherit via back propagation  FilterDenConstantOutMin=[]  FilterDenConstantOutMax=[]  PCopyOutDataTypeStr=Inherit: Inherit via back propagation  PCopyOutMin=[]  PCopyOutMax=[]  NCopyOutDataTypeStr=Inherit: Inherit via back propagation  NCopyOutMin=[]  NCopyOutMax=[]  IntegratorContinuousStateAttributes=''  IntegratorStateMustResolveToSignalObject=off  IntegratorRTWStateStorageClass=Auto  FilterContinuousStateAttributes=''  FilterStateMustResolveToSignalObject=off  FilterRTWStateStorageClass=Auto  ParallelPVariant=InternalParameters  IdealPVariant=Disabled  IVariant=InternalParameters  DVariant=InternalParameters  IntegratorVariant=Discrete  SatVariant=Disabled  AWVariant=Passthrough  PCopyVariant=Disabled  TRVariant=Disabled  FdbkBlocksVariant=Forward  IdealPFdbkVariant=Disabled  SatFdbkVariant=Disabled  DerivativeFilterVariant=ForwardEulerFilter  NVariant=InternalParameters  NCopyVariant=Disabled  FilterICVariant=InternalICsFilter  IntegratorICVariant=InternalICs  ExternalResetVariant=Disabled  TRSumVariant=Passthrough  SumFdbkVariant=Disabled  SumVariant=Sum_PID  TsampFilterVariant=InternalTs  TsampNgainVariant=Passthrough  TsampIntegralVariant=Disabled_SignalSpec  ExternalSaturationOutDataTypeStr=Inherit: Same as second input
  Publish1 : robotlib/Publish  topicSource=Select from ROS network  topic=/ackermann_steering_controller/cmd_vel  messageType=geometry_msgs/Twist  legacyBusStruct=off  messageQueueLength=1
  Pure Pursuit : robotalgslib/Pure Pursuit  DesiredLinearVelocity=1.5  MaxAngularVelocity=2  LookaheadDistance=1.3  TargetDirPort=on  SimulateUsing=Code generation
      settings: LibrarySourceBlock=navlib/Control Algorithms/Pure Pursuit
  Sum2 : Sum  Inputs=|+-
  Terminator : Terminator
  Tune_after : Scope  NumInputPorts=2
  Tune_before : Scope  NumInputPorts=2
  Zero2 : Constant  Commented=on  Value=0  OutDataTypeStr=Inherit: Inherit via back propagation
  wires:
  Pose/1 -> Pure Pursuit/1
  Waypoints/1 -> Pure Pursuit/2
  Bus Assignment1/1 -> Publish1/1
  Blank Message1/1 -> Bus Assignment1/1
  Pure Pursuit/3 -> Terminator/1
  Pure Pursuit/1 -> Tune_after/1, Tune_before/1, Sum2/1  "Ref"
  Pure Pursuit/2 -> Bus Assignment1/3
  In3/1 -> Tune_before/2, Sum2/2
  Sum2/1 -> PID Controller/1
  PID Controller/1 -> Tune_after/2, Bus Assignment1/2
  Zero2/1 -> Manual Switch2/1
  PID Controller3/1 -> Closed-Loop PID Autotuner2/1
  Manual Switch2/1 -> Closed-Loop PID Autotuner2/3
  Closed-Loop PID Autotuner2/3 -> Display4/1
  Closed-Loop PID Autotuner2/2 -> Display6/1
  One2/1 -> Manual Switch2/2

== system Hunter_gazebo_call/old version/Generate New Path  ==
  Pose : Inport
  Action Port : ActionPort  PropagateVarSize=During execution  ActionPortLabel=if(u1 == 0 | u2 == 0)
  Generate New Waypoint : Subsystem
  Subscribe : robotlib/Subscribe  topicSource=Select from ROS network  topic=/lidar  messageType=sensor_msgs/PointCloud2  SampleTime=-1  legacyBusStruct=off  messageQueueLength=1
  Subsystem : Subsystem  Commented=on
  generate_odomWaypoints : MATLAB Function  TreatAsAtomicUnit=on
  odomWP : Outport
  wires:
  Subscribe/2 -> Generate New Waypoint/1(rawData)
  Subscribe/1 -> Generate New Waypoint/Enable
  Pose/1 -> generate_odomWaypoints/1(pose)
  generate_odomWaypoints/1(odomWaypoints) -> odomWP/1
  Generate New Waypoint/1(waypoints) -> generate_odomWaypoints/2(waypoints)

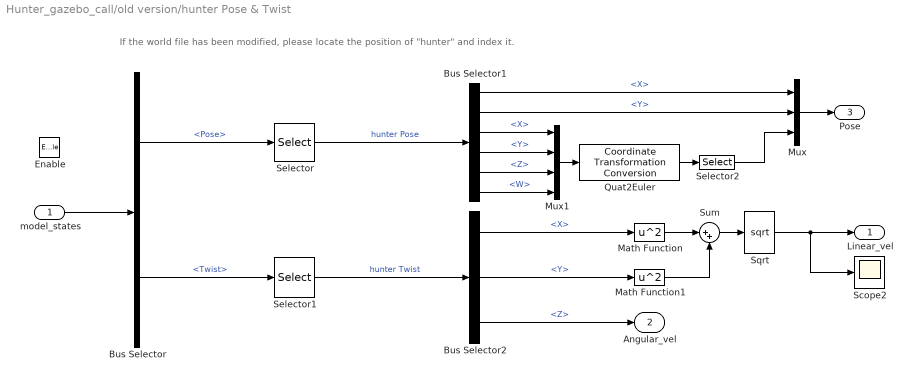
== system Hunter_gazebo_call/old version/hunter Pose & Twist ==
  note: If the world file has been modified, please locate the position of "hunter" and index it.
  model_states : Inport
  Enable : EnablePort  StatesWhenEnabling=reset
  Bus Selector : BusSelector  OutputSignals=Pose,Twist
  Bus Selector1 : BusSelector  OutputSignals=Position.X,Position.Y,Orientation.X,Orientation.Y,Orientation.Z,Orientation.W
  Bus Selector2 : BusSelector  OutputSignals=Linear.X,Linear.Y,Angular.Z
  Math Function : Math  Operator=square
  Math Function1 : Math  Operator=square
  Mux : Mux  Inputs=3
  Mux1 : Mux
  Quat2Euler : robotcorelib/Coordinate Transformation Conversion  InputRepresentation=Quaternion  InputEulerSequence=ZYX  ShowTrVecInputPort=on  OutputRepresentation=Euler Angles  OutputEulerSequence=ZYX  ShowTrVecOutputPort=on  SimulateUsing=Interpreted execution
  Scope2 : Scope
  Selector : Selector  InputPortWidth=350  IndexOptions=Index vector (dialog)  Indices=[137]  OutputSizes=1
  Selector1 : Selector  InputPortWidth=350  IndexOptions=Index vector (dialog)  Indices=[137]  OutputSizes=1
  Selector2 : Selector  InputPortWidth=3  IndexOptions=Index vector (dialog)  Indices=3  OutputSizes=1
  Sqrt : Sqrt
  Sum : Sum  Inputs=|++
  Linear_vel : Outport
  Angular_vel : Outport  Port=2
  Pose : Outport  Port=3
  wires:
  model_states/1 -> Bus Selector/1
  Bus Selector1/5 -> Mux1/3  "<Z>"
  Bus Selector1/3 -> Mux1/1  "<X>"
  Selector/1 -> Bus Selector1/1  "hunter Pose"
  Bus Selector1/6 -> Mux1/4  "<W>"
  Bus Selector2/1 -> Math Function/1  "<X>"
  Bus Selector1/4 -> Mux1/2  "<Y>"
  Selector1/1 -> Bus Selector2/1  "hunter Twist"
  Bus Selector1/1 -> Mux/1  "<X>"
  Bus Selector1/2 -> Mux/2  "<Y>"
  Bus Selector/1 -> Selector/1  "<Pose>"
  Bus Selector/2 -> Selector1/1  "<Twist>"
  Selector2/1 -> Mux/3
  Sum/1 -> Sqrt/1
  Bus Selector2/2 -> Math Function1/1  "<Y>"
  Math Function/1 -> Sum/1
  Math Function1/1 -> Sum/2
  Sqrt/1 -> Linear_vel/1, Scope2/1
  Bus Selector2/3 -> Angular_vel/1  "<Z>"
  Mux/1 -> Pose/1
  Mux1/1 -> Quat2Euler/1
  Quat2Euler/1 -> Selector2/1

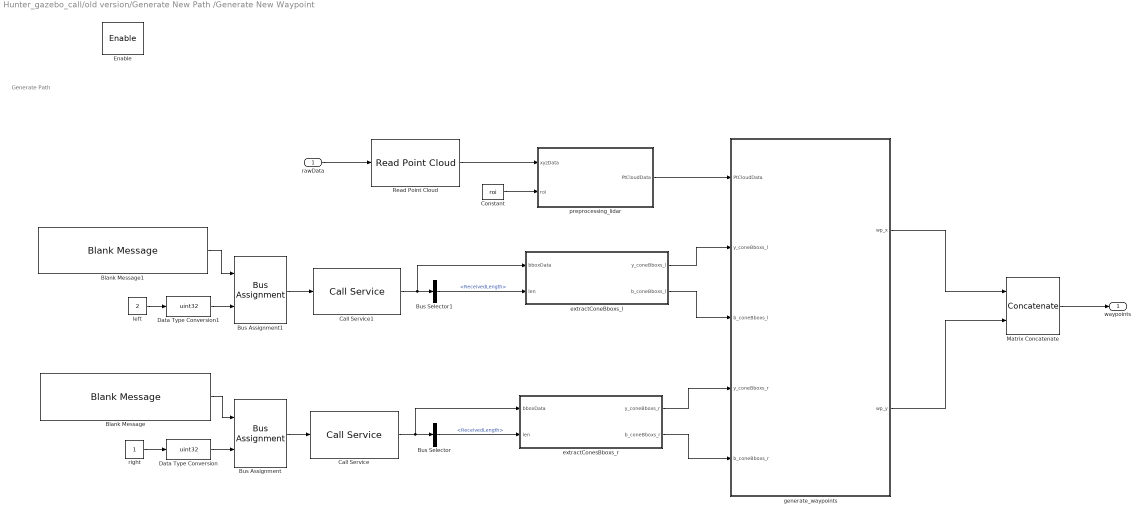
== system Hunter_gazebo_call/old version/Generate New Path /Generate New Waypoint ==
  note: Generate Path
  rawData : Inport
  Enable : EnablePort  PropagateVarSize=During execution
  Blank Message : robotlib/Blank Message  messageClass=Service Request  entityType=cob_object_detection_msgs/DetectObjects  messageType=cob_object_detection_msgs/DetectObjectsRequest  SampleTime=inf  legacyBusStruct=off
  Blank Message1 : robotlib/Blank Message  messageClass=Service Request  entityType=cob_object_detection_msgs/DetectObjects  messageType=cob_object_detection_msgs/DetectObjectsRequest  SampleTime=inf  legacyBusStruct=off
  Bus Assignment : BusAssignment  AssignedSignals=Roi.Height
  Bus Assignment1 : BusAssignment  AssignedSignals=Roi.Height
  Bus Selector : BusSelector  OutputSignals=ObjectList.Detections_SL_Info.ReceivedLength
  Bus Selector1 : BusSelector  OutputSignals=ObjectList.Detections_SL_Info.ReceivedLength
  Call Service : robotlib/Call Service  topicSource=Specify your own  service=/Activate_yolo  serviceType=cob_object_detection_msgs/DetectObjects  connectionTimeout=5  keepPersistent=off  ShowErrorCodeOutput=off  legacyBusStruct=off
  Call Service1 : robotlib/Call Service  topicSource=Specify your own  service=/Activate_yolo  serviceType=cob_object_detection_msgs/DetectObjects  connectionTimeout=5  keepPersistent=off  ShowErrorCodeOutput=off  legacyBusStruct=off
  Constant : Constant  Value=roi
  Data Type Conversion : DataTypeConversion  OutDataTypeStr=uint32  SaturateOnIntegerOverflow=off  RndMeth=Floor
  Data Type Conversion1 : DataTypeConversion  OutDataTypeStr=uint32  SaturateOnIntegerOverflow=off  RndMeth=Floor
  Matrix Concatenate : Concatenate  Mode=Multidimensional array  ConcatenateDimension=2
  Read Point Cloud : robotlib/Read Point Cloud  MaximumPointCloudSize=[1, 32768]  PreserveStructure=on  ShowRGBOutput=off  ShowIntensityOutput=off  ShowErrorCodeOutput=off  VariableSizeOutputs=off
  extractConeBboxs_l : MATLAB Function  TreatAsAtomicUnit=on
  extractConesBboxs_r : MATLAB Function  TreatAsAtomicUnit=on
  generate_waypoints : MATLAB Function  TreatAsAtomicUnit=on
  left : Constant  Value=2
  preprocessing_lidar : MATLAB Function  TreatAsAtomicUnit=on
  right : Constant
  waypoints : Outport
  wires:
  rawData/1 -> Read Point Cloud/1
  Read Point Cloud/1 -> preprocessing_lidar/1(xyzData)
  Constant/1 -> preprocessing_lidar/2(roi)
  Call Service/1 -> extractConesBboxs_r/1(bboxData), Bus Selector/1
  right/1 -> Data Type Conversion/1
  Bus Assignment1/1 -> Call Service1/1
  Data Type Conversion/1 -> Bus Assignment/2
  Blank Message1/1 -> Bus Assignment1/1
  left/1 -> Data Type Conversion1/1
  Call Service1/1 -> extractConeBboxs_l/1(bboxData), Bus Selector1/1
  Bus Selector1/1 -> extractConeBboxs_l/2(len)  "<ReceivedLength>"
  Bus Selector/1 -> extractConesBboxs_r/2(len)  "<ReceivedLength>"
  Bus Assignment/1 -> Call Service/1
  Data Type Conversion1/1 -> Bus Assignment1/2
  Blank Message/1 -> Bus Assignment/1
  extractConeBboxs_l/1(y_coneBboxs_l) -> generate_waypoints/2(y_coneBboxs_l)
  extractConeBboxs_l/2(b_coneBboxs_l) -> generate_waypoints/3(b_coneBboxs_l)
  preprocessing_lidar/1(PtCloudData) -> generate_waypoints/1(PtCloudData)
  extractConesBboxs_r/1(y_coneBboxs_r) -> generate_waypoints/4(y_coneBboxs_r)
  extractConesBboxs_r/2(b_coneBboxs_r) -> generate_waypoints/5(b_coneBboxs_r)
  generate_waypoints/1(wp_x) -> Matrix Concatenate/1
  generate_waypoints/2(wp_y) -> Matrix Concatenate/2
  Matrix Concatenate/1 -> waypoints/1

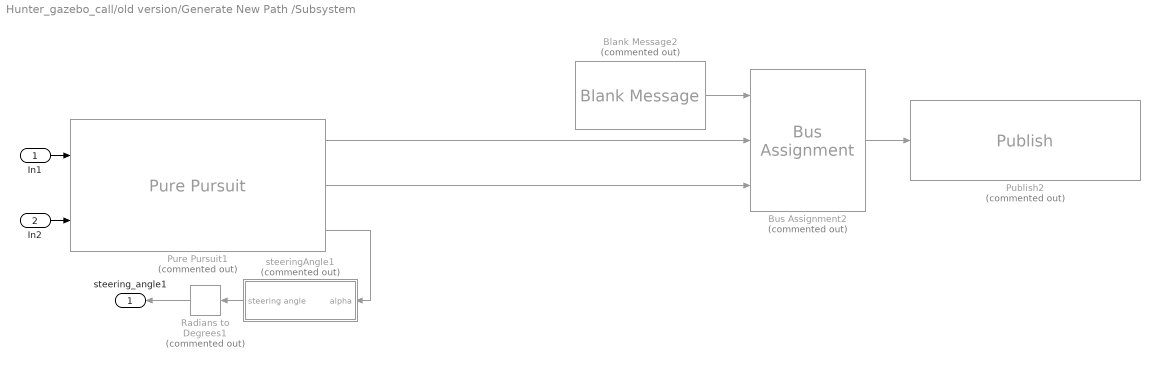
== system Hunter_gazebo_call/old version/Generate New Path /Subsystem ==
  In1 : Inport
  In2 : Inport  Port=2
  Blank Message2 : robotlib/Blank Message  Commented=on  messageClass=Message  entityType=geometry_msgs/Twist  messageType=geometry_msgs/Twist  SampleTime=inf  legacyBusStruct=off
  Bus Assignment2 : BusAssignment  Commented=on  AssignedSignals=Linear.X,Angular.Z
  Publish2 : robotlib/Publish  Commented=on  topicSource=Select from ROS network  topic=/ackermann_steering_controller/cmd_vel  messageType=geometry_msgs/Twist  legacyBusStruct=off  messageQueueLength=1
  Pure Pursuit1 : robotalgslib/Pure Pursuit  Commented=on  DesiredLinearVelocity=1.5  MaxAngularVelocity=2  LookaheadDistance=1.3  TargetDirPort=on  SimulateUsing=Code generation
      settings: LibrarySourceBlock=navlib/Control Algorithms/Pure Pursuit
  Radians to Degrees1 : simulink_extras/Transformations/Radians to Degrees  Commented=on
  steeringAngle1 : Subsystem  Commented=on
  steering_angle1 : Outport
  wires:
  Pure Pursuit1/1 -> Bus Assignment2/2
  Bus Assignment2/1 -> Publish2/1
  Pure Pursuit1/3 -> steeringAngle1/1(alpha)
  Pure Pursuit1/2 -> Bus Assignment2/3
  steeringAngle1/1(steering angle) -> Radians to Degrees1/1
  Radians to Degrees1/1 -> steering_angle1/1
  In1/1 -> Pure Pursuit1/1
  Blank Message2/1 -> Bus Assignment2/1
  In2/1 -> Pure Pursuit1/2

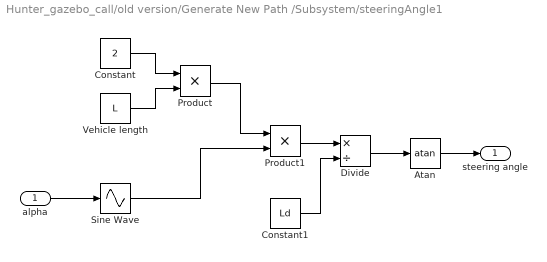
== system Hunter_gazebo_call/old version/Generate New Path /Subsystem/steeringAngle1 ==
  alpha : Inport
  Atan : Trigonometry  Operator=atan
  Constant : Constant  Value=2
  Constant1 : Constant  Value=Ld
  Divide : Product  Inputs=*/
  Product : Product
  Product1 : Product
  Sine Wave : Sin  TimeSource=Use external signal  SampleTime=0
  Vehicle length : Constant  Value=L
  steering angle : Outport
  wires:
  Constant/1 -> Product/1
  Vehicle length/1 -> Product/2
  alpha/1 -> Sine Wave/1
  Product/1 -> Product1/1
  Sine Wave/1 -> Product1/2
  Product1/1 -> Divide/1
  Constant1/1 -> Divide/2
  Divide/1 -> Atan/1
  Atan/1 -> steering angle/1

== matlab function Hunter_gazebo_call/Generate New Path /Generate New Waypoint/generate_waypoints ==
  data: PtCloudData input single size=[3000 3]; y_coneBboxs_l input; b_coneBboxs_l input; y_coneBboxs_r input; b_coneBboxs_r input; wp_x output size=[50,1]; wp_y output size=[50,1]
function [wp_x, wp_y] = generate_waypoints(PtCloudData, y_coneBboxs_l, b_coneBboxs_l,y_coneBboxs_r, b_coneBboxs_r)      
    %#codegen
    coder.extrinsic("generateWaypoints");
    wp_x = double(zeros(50,1));
    wp_y = double(zeros(50,1));

    [wp_x, wp_y] = generateWaypoints(PtCloudData,...
                                     y_coneBboxs_l, b_coneBboxs_l,...
                                     y_coneBboxs_r, b_coneBboxs_r);
end

== matlab function Hunter_gazebo_call/Generate New Path /Generate New Waypoint/preprocessing_lidar ==
  data: xyzData input single; PtCloudData output size=[3000 3]
function PtCloudData = preprocessing_lidar(xyzData)
    % waypoint_x, waypoint_y
    %% preprocessing raw lidar data
    params = lidarParameters('OS1Gen1-64',512);
    roi = [0, 7, -7, 7, -1, 2];

    ptCloud = pointCloud(xyzData);
    ptCloudOrg = pcorganize(ptCloud,params);
    
    groundPtIdx = segmentGroundFromLidarData(ptCloudOrg);
    nonGroundPtCloud = select(ptCloudOrg,~groundPtIdx,'OutputSize','full');
    
    indices = findPointsInROI(nonGroundPtCloud,roi);
    roiPtCloud = select(nonGroundPtCloud,indices);

    roiPtCloud = pcdenoise(roiPtCloud,"PreserveStructure",true);
    PtCloudData = roiPtCloud.Location;
    
end

== matlab function Hunter_gazebo_call/Generate New Path /generate_odomWaypoints ==
  data: pose input; waypoints input; odomWaypoints output double size=[50,2]
function odomWaypoints = fcn(pose, waypoints)
    % pose [3x1] 
    % waypoints [1x2]
    
    % Initialize transformed waypoints
    odomWaypoints = zeros(size(waypoints));
    % odomWaypoints = zeros(3,2);
    
    % Extract the vehicle's yaw angle
    theta = pose(3);

    % Create the 2D rotation matrix
    R = [cos(theta), -sin(theta);
         sin(theta), cos(theta)];

    % Transform each waypoint
    for i = 1:size(waypoints,1)
        % Rotate the waypoint considering the vehicle's yaw
        rotatedPoint = R * waypoints(i,:)';

        % Translate considering the vehicle's position in the odom frame
        odomWaypoints(i,:) = rotatedPoint' + pose(1:2)';
    end
    
    
end

== matlab function Hunter_gazebo_call/GenerateWP Logic/checkFirstRun ==
  data: odomWP input; u1 output
function u1 = checkWP(odomWP)
    
        
    if isempty(find(odomWP)) 
        u1 = 0;  % generate new waypoint
    else
        u1 = 1;  % follow existing waypoint
    end

end

== matlab function Hunter_gazebo_call/GenerateWP Logic/checkSecondRun ==
  data: odomWP input; u2 output; currentPose input
function u2 = checkDist(odomWP, currentPose)

   if norm(odomWP(end,:) - [currentPose(1) currentPose(2)]) < 2
       u2 = 0;  % generate new waypoints
   else
       u2 = 1;  % follow existing waypoints
   end

== matlab function Hunter_gazebo_call/old version/Generate New Path /generate_odomWaypoints ==
  data: pose input; waypoints input; odomWaypoints output double size=[50,2]
function odomWaypoints = fcn(pose, waypoints)
    % Initialize transformed waypoints
    odomWaypoints = zeros(size(waypoints));
    % odomWaypoints = zeros(3,2);
    
    % Extract the vehicle's yaw angle
    theta = pose(3);

    % Create the 2D rotation matrix
    R = [cos(theta), -sin(theta);
         sin(theta), cos(theta)];

    % Transform each waypoint
    for i = 1:size(waypoints,1)
        % Rotate the waypoint considering the vehicle's yaw
        rotatedPoint = R * waypoints(i,:)';

        % Translate considering the vehicle's position in the odom frame
        odomWaypoints(i,:) = rotatedPoint' + pose(1:2)';
    end
    
    
end

== matlab function Hunter_gazebo_call/old version/Generate New Path /Generate New Waypoint/extractConesBboxs_r ==
  data: y_coneBboxs_r output size=[50 4]; bboxData input; len input; b_coneBboxs_r output size=[50 4]
function [y_coneBboxs_r,b_coneBboxs_r] = extractConesBboxs_r(bboxData, len)

    temp_y_coneBboxs = zeros(len,4);
    temp_b_coneBboxs = zeros(len,4);

    y_count = 0;
    b_count = 0;

    % disp(len)
    for i = 1:len
        x = bboxData.ObjectList.Detections(i).Mask.Roi.X;
        y = bboxData.ObjectList.Detections(i).Mask.Roi.Y;
        w = bboxData.ObjectList.Detections(i).Mask.Roi.Width;
        h = bboxData.ObjectList.Detections(i).Mask.Roi.Height;

        label = char(bboxData.ObjectList.Detections(i).Label)';
        label = label(:,1:6);
        
        if strcmp(label,'y_cone')
            y_count = y_count + 1;
            temp_y_coneBboxs(y_count,:) = [x y w h];
        elseif strcmp(label,'b_cone')
            b_count = b_count + 1;
            temp_b_coneBboxs(b_count,:) = [x y w h];
        else
            disp("No");
        end
    end
   
    y_coneBboxs_r = temp_y_coneBboxs(1:y_count, :);
    b_coneBboxs_r = temp_b_coneBboxs(1:b_count, :);
   
end

== matlab function Hunter_gazebo_call/old version/Generate New Path /Generate New Waypoint/preprocessing_lidar ==
  data: xyzData input single; roi input; PtCloudData output size=[3000 3]
function PtCloudData = preprocessing_lidar(xyzData,roi)
    % waypoint_x, waypoint_y
    %% preprocessing raw lidar data
    params = lidarParameters('OS1Gen1-64',512);

    ptCloud = pointCloud(xyzData);
    ptCloudOrg = pcorganize(ptCloud,params);
    
    groundPtIdx = segmentGroundFromLidarData(ptCloudOrg);
    nonGroundPtCloud = select(ptCloudOrg,~groundPtIdx,'OutputSize','full');
    
    indices = findPointsInROI(nonGroundPtCloud,roi);
    roiPtCloud = select(nonGroundPtCloud,indices);

    roiPtCloud = pcdenoise(roiPtCloud,"PreserveStructure",true);
    PtCloudData = roiPtCloud.Location;
    
end

== matlab function Hunter_gazebo_call/Generate New Path /Generate New Waypoint/extractConeBboxs_l ==
  data: y_coneBboxs_l output size=[50 4]; bboxData input; len input; b_coneBboxs_l output size=[50 4]
function [y_coneBboxs_l, b_coneBboxs_l] = extractConesBboxs_l(bboxData, len)

    temp_y_coneBboxs = zeros(len,4);
    temp_b_coneBboxs = zeros(len,4);

    y_count = 0;
    b_count = 0;

    % disp(len)
    for i = 1:len
        x = bboxData.ObjectList.Detections(i).Mask.Roi.X;
        y = bboxData.ObjectList.Detections(i).Mask.Roi.Y;
        w = bboxData.ObjectList.Detections(i).Mask.Roi.Width;
        h = bboxData.ObjectList.Detections(i).Mask.Roi.Height;

        label = char(bboxData.ObjectList.Detections(i).Label)';
        label = label(:,1:6);
        
        if strcmp(label,'y_cone')
            y_count = y_count + 1;
            temp_y_coneBboxs(y_count,:) = [x y w h];
        elseif strcmp(label,'b_cone')
            b_count = b_count + 1;
            temp_b_coneBboxs(b_count,:) = [x y w h];
        else
            disp("No");
        end
    end
   
    y_coneBboxs_l = temp_y_coneBboxs(1:y_count, :);
    b_coneBboxs_l = temp_b_coneBboxs(1:b_count, :);
   
end
